simulink model "pendulo_invertido_bloques"  (R2025a)
settings: Solver=ode45  StartTime=0.0  StopTime=10.0  RelTol=1e-3
PreLoadFcn:
  | % Parámetros físicos
  | Ip   = 0.0079;     % kg*m^2
  | Mc   = 0.7031;     % kg
  | lp   = 0.3302;     % m
  | lp2  = lp^2;       % m^2
  | lp3  = lp^3;       % m^3
  | Mp   = 0.23;       % kg
  | Mp2  = Mp^2;       % kg^2
  | Fc   = 0;          % N
  | Beq  = 4.3;        % Ns/m
  | g    = 9.81;       % m/s^2
  | Bp   = 0.0024;     % Nms/rad
  | 
  | % Condiciones iniciales de los estados
  | x       = 0;          % m
  | xdot      = 0;          % m/s
  | alpha   = 1*pi/180;   % rad
  | adot     = 0;          % rad/s
settings Model: Creator=Chris  LastModifiedBy=Chris

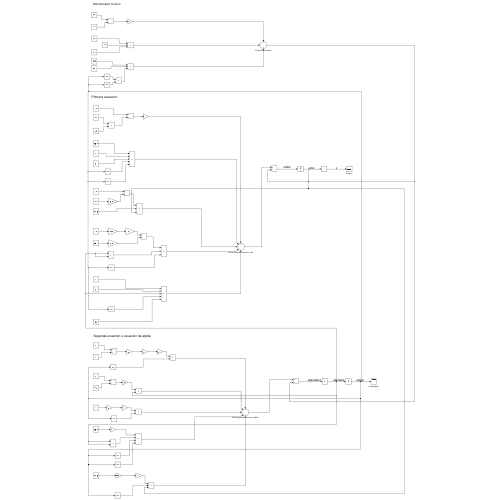
[thumbnail: Simulink's stored preview of the top-level diagram]
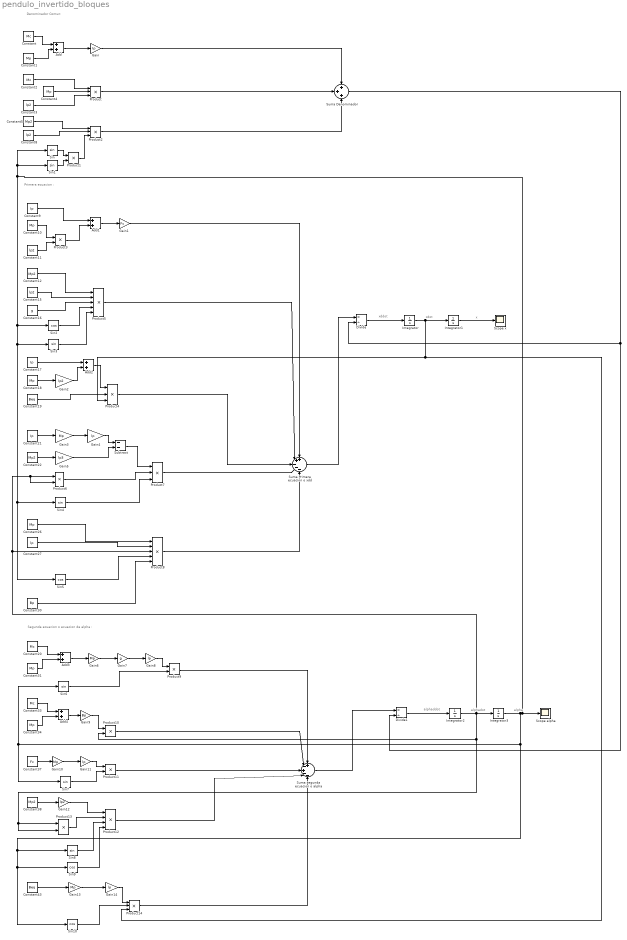
== system pendulo_invertido_bloques ==
  note: xddot
  note: Primera ecuacion :
  note: Denominador Comun:
  note: xdot
  note: x
  note: Segunda ecuacion o ecuacion de alpha :
  note: alphaddot
  note: alphadot
  note: alpha
  Add{,1..4} (5 alike) : Sum
  Constant{,2,20,33} (4 alike) : Constant  Value=Mc
  Constant{1,4,10,18,26,31,34} (7 alike) : Constant  Value=Mp
  Constant{3,8,11,15} (4 alike) : Constant  Value=lp2
  Constant{5,12,22,38} (4 alike) : Constant  Value=Mp2
  Constant16 : Constant  Value=g
  Constant17 : Constant  Value=Ip
  Constant19 : Constant  Value=Beq
  Constant21 : Constant  Value=Ip
  Constant27 : Constant  Value=lp
  Constant30 : Constant  Value=Bp
  Constant37 : Constant  Value=Fc
  Constant43 : Constant  Value=Beq
  Constant9 : Constant  Value=Ip
  Divide : Product  Inputs=*/
  Divide1 : Product  Inputs=*/
  Gain : Gain  Gain=Ip
  Gain1 : Gain  Gain=Fc
  Gain{3,6,10,13} (4 alike) : Gain  Gain=Mp
  Gain{4,8,11,14} (4 alike) : Gain  Gain=lp
  Gain12 : Gain  Gain=lp2
  Gain2 : Gain  Gain=lp2
  Gain5 : Gain  Gain=lp3
  Gain7 : Gain  Gain=g
  Gain9 : Gain  Gain=Bp
  Integrator : Integrator  InitialCondition=xdot
  Integrator1 : Integrator  InitialCondition=x
  Integrator2 : Integrator  InitialCondition=adot
  Integrator3 : Integrator  InitialCondition=alpha
  Product{,2,4,7,14} (5 alike) : Product  Inputs=3
  Product{1,3,6,9..11,13} (7 alike) : Product
  Product12 : Product  Inputs=4
  Product5 : Product  Inputs=5
  Product8 : Product  Inputs=5
  Scope alpha : Scope
      settings: ActiveDisplayYMinimum=-53.255338758236832  ActiveDisplayYMaximum=479.472581749331
  Scope x : Scope
      settings: ActiveDisplayYMinimum=-0.022885634637408558  ActiveDisplayYMaximum=0.26900712735939025
  Sin{,1,3..4,6..8} (7 alike) : Trigonometry
  Sin{2,5,9..10} (4 alike) : Trigonometry  Operator=cos
  Subtract : Sum  Inputs=--
  Suma Denominador : Sum  Inputs=+++
  Suma Primera ecuacion o xdd : Sum  Inputs=++---
  Suma segunda ecuacion o alpha : Sum  Inputs=+-+--
  wires:
  Constant/1 -> Add/1
  Constant1/1 -> Add/2
  Add/1 -> Gain/1
  Gain/1 -> Suma Denominador/1
  Constant4/1 -> Product/2
  Constant2/1 -> Product/1
  Constant3/1 -> Product/3
  Product/1 -> Suma Denominador/2
  Sin1/1 -> Product1/2
  Sin/1 -> Product1/1
  Product1/1 -> Product2/3
  Constant8/1 -> Product2/2
  Constant5/1 -> Product2/1
  Product2/1 -> Suma Denominador/3
  Constant9/1 -> Add1/1
  Constant10/1 -> Product3/1
  Constant11/1 -> Product3/2
  Product3/1 -> Add1/2
  Add1/1 -> Gain1/1
  Gain1/1 -> Suma Primera ecuacion o xdd/1
  Constant12/1 -> Product5/1
  Constant15/1 -> Product5/2
  Constant16/1 -> Product5/3
  Sin2/1 -> Product5/4
  Sin3/1 -> Product5/5
  Product5/1 -> Suma Primera ecuacion o xdd/2
  Constant18/1 -> Gain2/1
  Constant17/1 -> Add2/1
  Gain2/1 -> Add2/2
  Add2/1 -> Product4/1
  Constant19/1 -> Product4/2
  Product4/1 -> Suma Primera ecuacion o xdd/3
  Constant21/1 -> Gain3/1
  Gain3/1 -> Gain4/1
  Constant22/1 -> Gain5/1
  Gain4/1 -> Subtract/1
  Gain5/1 -> Subtract/2
  Subtract/1 -> Product7/1
  Product6/1 -> Product7/2
  Sin4/1 -> Product7/3
  Product7/1 -> Suma Primera ecuacion o xdd/4
  Constant26/1 -> Product8/1
  Constant27/1 -> Product8/2
  Sin5/1 -> Product8/4
  Constant30/1 -> Product8/5
  Product8/1 -> Suma Primera ecuacion o xdd/5
  Integrator1/1 -> Scope x/1
  Suma Primera ecuacion o xdd/1 -> Divide/1
  Divide/1 -> Integrator/1
  Constant20/1 -> Add3/1
  Constant31/1 -> Add3/2
  Add3/1 -> Gain6/1
  Gain6/1 -> Gain7/1
  Gain7/1 -> Gain8/1
  Sin6/1 -> Product9/2
  Gain8/1 -> Product9/1
  Product9/1 -> Suma segunda ecuacion o alpha/1
  Constant33/1 -> Add4/1
  Constant34/1 -> Add4/2
  Add4/1 -> Gain9/1
  Gain9/1 -> Product10/1
  Product10/1 -> Suma segunda ecuacion o alpha/2
  Constant37/1 -> Gain10/1
  Gain10/1 -> Gain11/1
  Sin7/1 -> Product11/2
  Gain11/1 -> Product11/1
  Product11/1 -> Suma segunda ecuacion o alpha/3
  Constant38/1 -> Gain12/1
  Gain12/1 -> Product12/1
  Integrator3/1 -> Sin5/1, Sin4/1, Sin3/1, Sin2/1, Sin1/1, Sin/1, Scope alpha/1, Sin8/1, Sin9/1, Sin10/1, Sin6/1, Sin7/1
  Integrator2/1 -> Product13/2, Product13/1, Product10/2, Product8/3, Product6/2, Product6/1, Integrator3/1
  Product13/1 -> Product12/2
  Sin8/1 -> Product12/3
  Sin9/1 -> Product12/4
  Product12/1 -> Suma segunda ecuacion o alpha/4
  Constant43/1 -> Gain13/1
  Gain13/1 -> Gain14/1
  Integrator/1 -> Integrator1/1, Product14/3, Product4/3
  Gain14/1 -> Product14/1
  Sin10/1 -> Product14/2
  Product14/1 -> Suma segunda ecuacion o alpha/5
  Suma Denominador/1 -> Divide/2, Divide1/2
  Suma segunda ecuacion o alpha/1 -> Divide1/1
  Divide1/1 -> Integrator2/1
